simulink model "ex4_5_sum"  (R2020b)
settings: Solver=VariableStepAuto  StartTime=0.0  StopTime=0.04096  RelTol=1e-3
settings Model: Creator=seojoon  LastModifiedBy=seojoon

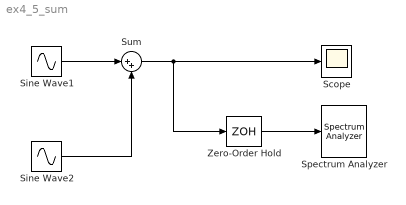
== system ex4_5_sum ==
  Scope : Scope
  Sine Wave1 : Sin  Amplitude=10  Frequency=2*pi*1000  SampleTime=0
  Sine Wave2 : Sin  Frequency=2*pi*500  SampleTime=0
  Spectrum Analyzer : SpectrumAnalyzer
  Sum : Sum  Inputs=|++
  Zero-Order Hold : ZeroOrderHold  SampleTime=1e-5
  wires:
  Zero-Order Hold/1 -> Spectrum Analyzer/1
  Sine Wave1/1 -> Sum/1
  Sine Wave2/1 -> Sum/2
  Sum/1 -> Zero-Order Hold/1, Scope/1
